simulink model "MBD_Week2_Prob2"  (R2020a)
settings: Solver=VariableStepAuto  StartTime=0.0  StopTime=10.0  RelTol=1e-3
undefined symbols (not defined in the file or in its folder): be, bv, le, lv
settings Model: Creator=Noel Varghese  LastModifiedBy=Noel Varghese

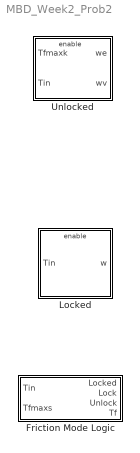
== system MBD_Week2_Prob2 ==
  Friction Mode Logic : Subsystem
  Locked : Subsystem
  Unlocked : Subsystem

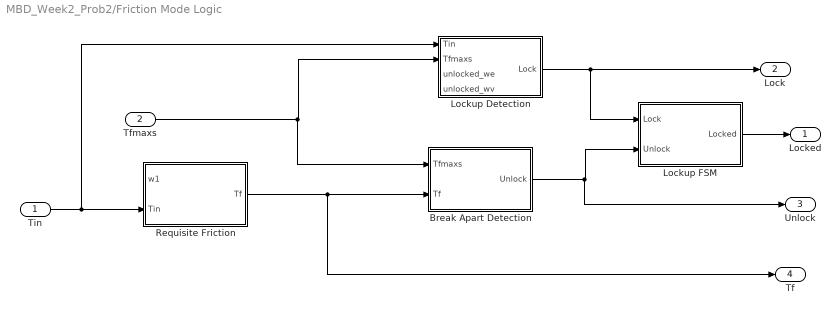
== system MBD_Week2_Prob2/Friction Mode Logic ==
  Tin : Inport
  Tfmaxs : Inport  Port=2
  Break Apart Detection : Subsystem
  Lockup Detection : Subsystem
  Lockup FSM : Subsystem
  Requisite Friction : Subsystem
  Locked : Outport
  Lock : Outport  Port=2
  Unlock : Outport  Port=3
  Tf : Outport  Port=4
  wires:
  Tin/1 -> Lockup Detection/1(Tin), Requisite Friction/2(Tin)
  Tfmaxs/1 -> Break Apart Detection/1(Tfmaxs), Lockup Detection/2(Tfmaxs)
  Requisite Friction/1(Tf) -> Tf/1, Break Apart Detection/2(Tf)
  Break Apart Detection/1(Unlock) -> Unlock/1, Lockup FSM/2(Unlock)
  Lockup Detection/1(Lock) -> Lock/1, Lockup FSM/1(Lock)
  Lockup FSM/1(Locked) -> Locked/1

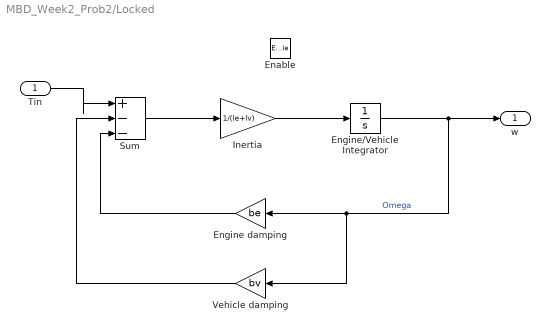
== system MBD_Week2_Prob2/Locked ==
  Tin : Inport
  Enable : EnablePort  StatesWhenEnabling=reset
  Engine damping : Gain  Gain=be
  Engine/Vehicle Integrator : Integrator
  Inertia : Gain  Gain=1/(le+lv)
  Sum : Sum  Inputs=|+--
  Vehicle damping : Gain  Gain=bv
  w : Outport
  wires:
  Vehicle damping/1 -> Sum/2
  Tin/1 -> Sum/1
  Engine/Vehicle Integrator/1 -> w/1, Vehicle damping/1, Engine damping/1  "Omega"
  Sum/1 -> Inertia/1
  Inertia/1 -> Engine/Vehicle Integrator/1
  Engine damping/1 -> Sum/3

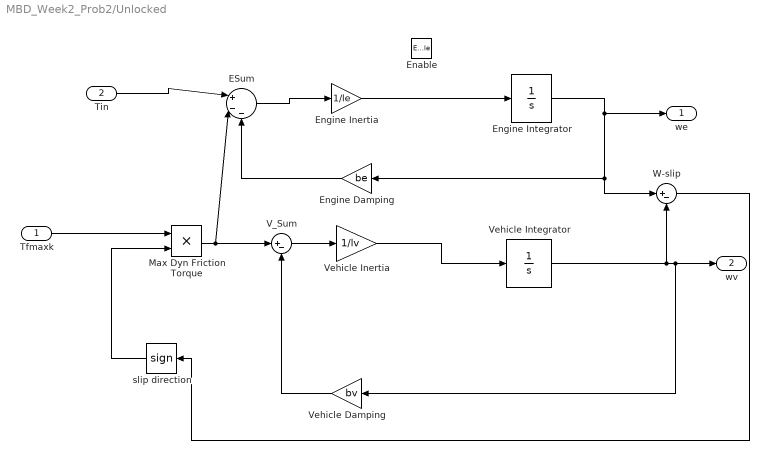
== system MBD_Week2_Prob2/Unlocked ==
  Tfmaxk : Inport
  Tin : Inport  Port=2
  Enable : EnablePort  StatesWhenEnabling=reset
  ESum : Sum  Inputs=|+--
  Engine Damping : Gain  Gain=be
  Engine Inertia : Gain  Gain=1/le
  Engine Integrator : Integrator
  Max Dyn Friction Torque : Product
  V_Sum : Sum  Inputs=|+-
  Vehicle Damping : Gain  Gain=bv
  Vehicle Inertia : Gain  Gain=1/lv
  Vehicle Integrator : Integrator
  W-slip : Sum  Inputs=|+-
  slip direction : Signum
  we : Outport
  wv : Outport  Port=2
  wires:
  slip direction/1 -> Max Dyn Friction Torque/2
  Max Dyn Friction Torque/1 -> ESum/2, V_Sum/1
  Vehicle Inertia/1 -> Vehicle Integrator/1
  Engine Integrator/1 -> we/1, W-slip/1, Engine Damping/1
  V_Sum/1 -> Vehicle Inertia/1
  Engine Inertia/1 -> Engine Integrator/1
  Vehicle Damping/1 -> V_Sum/2
  Tfmaxk/1 -> Max Dyn Friction Torque/1
  Tin/1 -> ESum/1
  Vehicle Integrator/1 -> wv/1, Vehicle Damping/1, W-slip/2
  W-slip/1 -> slip direction/1
  ESum/1 -> Engine Inertia/1
  Engine Damping/1 -> ESum/3

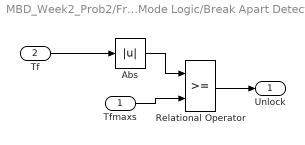
== system MBD_Week2_Prob2/Friction Mode Logic/Break Apart Detection ==
  Tfmaxs : Inport
  Tf : Inport  Port=2
  Abs : Abs
  Relational Operator : RelationalOperator  OutDataTypeStr=boolean  RndMeth=Simplest
  Unlock : Outport
  wires:
  Abs/1 -> Relational Operator/1
  Tf/1 -> Abs/1
  Tfmaxs/1 -> Relational Operator/2
  Relational Operator/1 -> Unlock/1

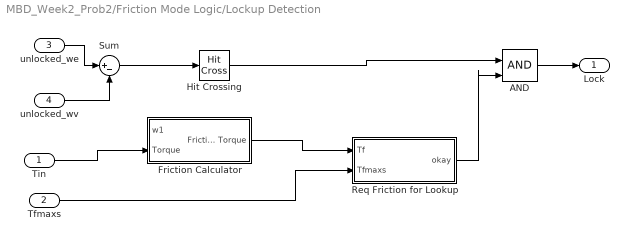
== system MBD_Week2_Prob2/Friction Mode Logic/Lockup Detection ==
  Tin : Inport
  Tfmaxs : Inport  Port=2
  unlocked_we : Inport  Port=3
  unlocked_wv : Inport  Port=4
  AND : Logic  IconShape=distinctive  AllPortsSameDT=off  OutDataTypeStr=boolean
  Friction Calculator : Subsystem
  Hit Crossing : HitCross
  Req Friction for Lookup : Subsystem
  Sum : Sum  Inputs=|+-
  Lock : Outport
  wires:
  Tin/1 -> Friction Calculator/2(Torque)
  Tfmaxs/1 -> Req Friction for Lookup/2(Tfmaxs)
  Friction Calculator/1(Friction Torque) -> Req Friction for Lookup/1(Tf)
  unlocked_we/1 -> Sum/1
  unlocked_wv/1 -> Sum/2
  Sum/1 -> Hit Crossing/1
  Hit Crossing/1 -> AND/1
  Req Friction for Lookup/1(okay) -> AND/2
  AND/1 -> Lock/1

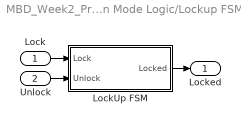
== system MBD_Week2_Prob2/Friction Mode Logic/Lockup FSM ==
  Lock : Inport
  Unlock : Inport  Port=2
  LockUp FSM : Subsystem
  Locked : Outport
  wires:
  Lock/1 -> LockUp FSM/1(Lock)
  Unlock/1 -> LockUp FSM/2(Unlock)
  LockUp FSM/1(Locked) -> Locked/1

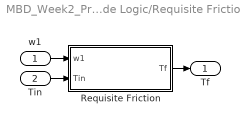
== system MBD_Week2_Prob2/Friction Mode Logic/Requisite Friction ==
  w1 : Inport
  Tin : Inport  Port=2
  Requisite Friction : Subsystem
  Tf : Outport
  wires:
  w1/1 -> Requisite Friction/1(w1)
  Tin/1 -> Requisite Friction/2(Tin)
  Requisite Friction/1(Tf) -> Tf/1

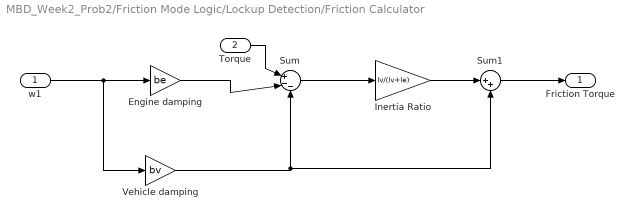
== system MBD_Week2_Prob2/Friction Mode Logic/Lockup Detection/Friction Calculator ==
  w1 : Inport
  Torque : Inport  Port=2
  Engine damping : Gain  Gain=be
  Inertia Ratio : Gain  Gain=lv/(lv+le)
  Sum : Sum  Inputs=|+--
  Sum1 : Sum  Inputs=|++
  Vehicle damping : Gain  Gain=bv
  Friction Torque : Outport
  wires:
  Vehicle damping/1 -> Sum1/2, Sum/3
  w1/1 -> Vehicle damping/1, Engine damping/1
  Sum/1 -> Inertia Ratio/1
  Sum1/1 -> Friction Torque/1
  Engine damping/1 -> Sum/2
  Torque/1 -> Sum/1
  Inertia Ratio/1 -> Sum1/1

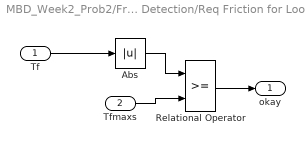
== system MBD_Week2_Prob2/Friction Mode Logic/Lockup Detection/Req Friction for Lookup ==
  Tf : Inport
  Tfmaxs : Inport  Port=2
  Abs : Abs
  Relational Operator : RelationalOperator  OutDataTypeStr=boolean  RndMeth=Simplest
  okay : Outport
  wires:
  Abs/1 -> Relational Operator/1
  Tf/1 -> Abs/1
  Tfmaxs/1 -> Relational Operator/2
  Relational Operator/1 -> okay/1

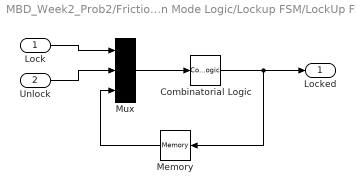
== system MBD_Week2_Prob2/Friction Mode Logic/Lockup FSM/LockUp FSM ==
  Lock : Inport
  Unlock : Inport  Port=2
  Combinatorial Logic : CombinatorialLogic  TruthTable=[0;1;0;0;1;1;1;0]
  Memory : Memory
  Mux : Mux  Inputs=3
  Locked : Outport
  wires:
  Lock/1 -> Mux/1
  Unlock/1 -> Mux/2
  Memory/1 -> Mux/3
  Mux/1 -> Combinatorial Logic/1
  Combinatorial Logic/1 -> Memory/1, Locked/1

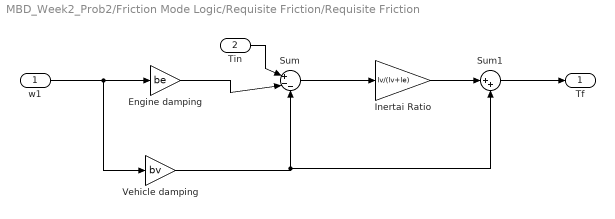
== system MBD_Week2_Prob2/Friction Mode Logic/Requisite Friction/Requisite Friction ==
  w1 : Inport
  Tin : Inport  Port=2
  Engine damping : Gain  Gain=be
  Inertai Ratio : Gain  Gain=lv/(lv+le)
  Sum : Sum  Inputs=|+--
  Sum1 : Sum  Inputs=|++
  Vehicle damping : Gain  Gain=bv
  Tf : Outport
  wires:
  Tin/1 -> Sum/1
  Engine damping/1 -> Sum/2
  Vehicle damping/1 -> Sum1/2, Sum/3
  Sum/1 -> Inertai Ratio/1
  Inertai Ratio/1 -> Sum1/1
  Sum1/1 -> Tf/1
  w1/1 -> Vehicle damping/1, Engine damping/1
